simulink model "Accelerate"  (R2018a)
settings: Solver=ode113  StartTime=0.0  StopTime=20  RelTol=1e-3
settings Model: Creator=28718  LastModifiedBy=28718

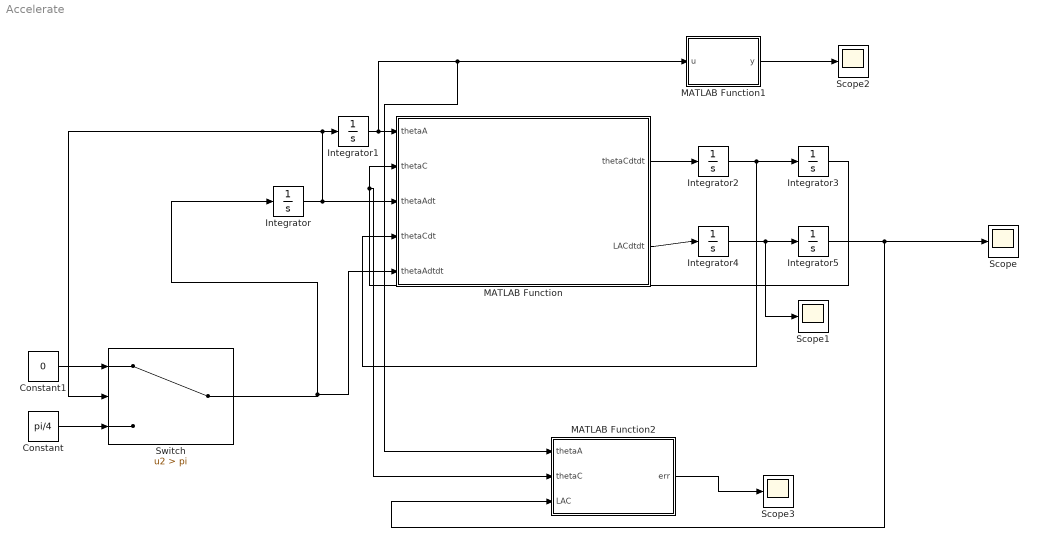
== system Accelerate ==
  Constant : Constant  Value=pi/4
  Constant1 : Constant  Value=0
  Integrator{,1..4} (5 alike) : Integrator
  Integrator5 : Integrator  InitialCondition=5
  MATLAB Function : MATLAB Function  TreatAsAtomicUnit=on
  MATLAB Function1 : MATLAB Function  TreatAsAtomicUnit=on
  MATLAB Function2 : MATLAB Function  TreatAsAtomicUnit=on
  Scope{,1..3} (4 alike) : Scope
  Switch : Switch  Criteria=u2 > Threshold  Threshold=pi
  wires:
  Integrator/1 -> Switch/2, Integrator1/1, MATLAB Function/3(thetaAdt)
  Integrator1/1 -> MATLAB Function2/1(thetaA), MATLAB Function1/1(u), MATLAB Function/1(thetaA)
  MATLAB Function/1(thetaCdtdt) -> Integrator2/1
  Integrator2/1 -> Integrator3/1, MATLAB Function/4(thetaCdt)
  Integrator3/1 -> MATLAB Function2/2(thetaC), MATLAB Function/2(thetaC)
  MATLAB Function/2(LACdtdt) -> Integrator4/1
  Integrator4/1 -> Scope1/1, Integrator5/1
  Integrator5/1 -> MATLAB Function2/3(LAC), Scope/1
  Constant1/1 -> Switch/1
  Constant/1 -> Switch/3
  Switch/1 -> MATLAB Function/5(thetaAdtdt), Integrator/1
  MATLAB Function1/1(y) -> Scope2/1
  MATLAB Function2/1(err) -> Scope3/1

== matlab function Accelerate/MATLAB Function1 ==
  data: u input; y output
function y = fcn(u)
n=round(u/(2*pi));  %通过四舍五入函数算的这个2pi的几个整数倍
y=u-n*2*pi;
end

== matlab function Accelerate/MATLAB Function ==
  data: thetaA input; thetaCdtdt output; thetaC input; thetaAdt input; thetaCdt input; thetaAdtdt input; LACdtdt output
function [thetaCdtdt,LACdtdt] = fcn(thetaA,thetaC,thetaAdt,thetaCdt,thetaAdtdt)

LAB=1;
LBC=4;

thetaCdtdt = (- LAB*sin(thetaA)*thetaAdt^2 + LBC*sin(thetaC)*thetaCdt^2 + LAB*thetaAdtdt*cos(thetaA))/(LBC*cos(thetaC));
LACdtdt = -(LBC*thetaCdt^2*cos(thetaC)^2 + LBC*thetaCdt^2*sin(thetaC)^2 + LAB*thetaAdt^2*cos(thetaA)*cos(thetaC) - LAB*thetaAdt^2*sin(thetaA)*sin(thetaC) + LAB*thetaAdtdt*cos(thetaA)*sin(thetaC) + LAB*thetaAdtdt*cos(thetaC)*sin(thetaA))/cos(thetaC);

== matlab function Accelerate/MATLAB Function2 ==
  data: thetaA input; err output; thetaC input; LAC input
function err = fcn(thetaA,thetaC,LAC)
LAB=1;
LBC=4;
errX=LAB * cos(thetaA) + LBC * cos(thetaC) - LAC;   %水平方向的位置误差
errY=LAB * sin(thetaA) - LBC * sin(thetaC);         %竖直方向的位置误差
err = sqrt(errX^2 + errY^2);    %如果直接用水平的误差加上竖直的误差可能一个0.5,一个-0.5抵消了
end
